simulink model "ev"  (R2021a)
settings: Solver=ode4  StartTime=0  StopTime=1082  FixedStep=sim_dt  RelTol=1e-3
model workspace (MAT data in the model file):
  T_eff_bp = [-270; -210; -150; -90; -30; 30; 90; 150; 210; 270]
  T_eff_bp_2 = [-270; -210; -150; -90; -30; 30; 90; 150; 210; 270]
  losses_table = [108927.107777 7820.2782368 7820.17609997 7820.2782368 7820.2782368 7820.2782368 7820.2782368 7820.26172359 7820.2782368 9345.38006027 108927.107777 7820.2782368 ... (100 elements, 10x10)]
  losses_table_2 = [108927.107777 7820.2782368 7820.17609997 7820.2782368 7820.2782368 7820.2782368 7820.2782368 7820.26172359 7820.2782368 9345.38006027 108927.107777 7820.2782368 ... (100 elements, 10x10)]
  w_eff_bp = [0; 888.888888889; 1777.77777778; 2666.66666667; 3555.55555556; 4444.44444444; 5333.33333333; 6222.22222222; 7111.11111111; 8000]
  w_eff_bp_2 = [0; 888.888888889; 1777.77777778; 2666.66666667; 3555.55555556; 4444.44444444; 5333.33333333; 6222.22222222; 7111.11111111; 8000]
undefined symbols (not defined in the file): Af, alpha, Bt, C, C_fa, C_free, C_sa_bat, C_sa_uc, Cd, Cmax, Continuous, Crr, DoD, effi, etaFD, etaG, FD, G, gear, Iucmax, m, M1m, M2m, Max, npar, npar_free, npara, nparf, nparfa, nparsa_bat, nparsa_UC, nser, nser_free, nserfa, nsersa_bat, nsersa_UC, Qbat, regenmax, Ri_BP, RL, ro, Rsc, Rsc_A, Rsc_F, Rsc_sa_bat, Rsc_sa_uc, rw, sim_dt, SOC_BP, SoCbatmax, SoCbatmin, SoCucmax, SoCucmin, speed, torque, VinBat, Voc_BP, Vuc, Vuc_fa, Vuc_free ... (+2)
libraries: autolibshared x41, simulink x26, autolibdcdc x13, autolibdatasheetbattery x7, autolibmappedmotor x6, fl_lib x3, nesl_utility x3, spsSupercapacitorLib x3, pid_lib x1
(part 7 of 18)

== system ev/Tesis/HESS/Battery model ==
  motor_pwr_contr : Inport
  Add : Sum  Inputs=+-
  Bus Selector : BusSelector  OutputSignals=BattSoc,BattCurr,BattPwr
  Compare To Constant1 : simulink/Logic and Bit Operations/Compare To Constant  relop=<=  const=0.2  OutDataTypeStr=boolean
  Constant2 : Constant  Value=293.15
  Current_calc : Product  Inputs=/*
  Datasheet Battery : autolibdatasheetbattery/Datasheet Battery  CapacityCtrl=Parameter  OutputVlt=Unfiltered  BattChargeMax=Qbat  Em=Voc_BP  CapLUTBp=SOC_BP  RInt=iR_bp  BattTempBp=Temp_bp  CapSOCBp=SOC_BP  Ns=nser  Np=npar  BattCapInit=Qbat*(1-DoD)  Tc=0.01  Vinit=3.3342*nser  RefBlkName='autolibdatasheetbattery/Datasheet Battery'
      settings: SourceProductBaseCode=PW
  Display1 : DisplayBlock  LabelPosition=Hide  Format=short  Transparency=1
  Gain4 : Gain  Gain=nser
  Gain5 : Gain  Gain=nser/npar
  MATLAB Function1 : MATLAB Function  TreatAsAtomicUnit=on
  Mux : Mux
  Mux12 : Mux  Inputs=2
  OCV1 : Lookup_n-D  NumberOfTableDimensions=1  BreakpointsForDimension1=SOC_BP  Table=Voc_BP  InternalRulePriority=Speed  RndMeth=Simplest  InputSameDT=on
  Product1 : Product
  Ri1 : Lookup_n-D  NumberOfTableDimensions=1  BreakpointsForDimension1=SOC_BP  Table=Ri_BP  InternalRulePriority=Speed  RndMeth=Simplest  InputSameDT=on
  Scope{1,5..7,13..14,26,39,44} (9 alike) : Scope
  Stop Simulation : Stop
  To Workspace9 : ToWorkspace  VariableName=Batt  SaveFormat=Structure With Time  SampleTime=-1
  <BattCurr> : Outport
  Voltage : Outport  Port=2
  wires:
  Bus Selector/2 -> <BattCurr>/1, Scope26/1, Product1/2  "<BattCurr>"
  Gain5/1 -> MATLAB Function1/1(Ri), Product1/1, Scope1/1
  Datasheet Battery/2 -> Voltage/1, Mux/2  "Voltage"
  Bus Selector/1 -> Compare To Constant1/1, Ri1/1, OCV1/1, Scope7/1  "<BattSoc>"
  Mux/1 -> Scope14/1
  Compare To Constant1/1 -> Scope5/1, Stop Simulation/1
  Gain4/1 -> Add/1, Mux/1, Current_calc/1
  OCV1/1 -> Gain4/1
  Bus Selector/3 -> Mux12/1  "<BattPwr>"
  Ri1/1 -> Gain5/1
  Add/1 -> Mux/3
  MATLAB Function1/1(Vb) -> Mux/4, Scope44/1
  Product1/1 -> Add/2
  Mux12/1 -> Scope39/1
  Datasheet Battery/1 -> Scope6/1, Bus Selector/1, To Workspace9/1
  Constant2/1 -> Datasheet Battery/2
  Current_calc/1 -> MATLAB Function1/2(Ib), Datasheet Battery/1, Scope13/1  "I_batt"
  motor_pwr_contr/1 -> Mux12/2, MATLAB Function1/3(Pmot), Current_calc/2

== system ev/Tesis/HESS/Battery with DC//DC ==
  motor_pwr_contr : Inport
  Add3 : Sum  Inputs=+-
  Bidirectional DC-DC2 : autolibdcdc/Bidirectional DC-DC  Tc=1/1000  Vinit=320  Plimit=100000  param_loss=Single efficiency measurement  eff=100  v_loss_bp=[0 200 400 600 800 1000]  i_loss_bp=[0 25 50 75 100]  losses_table=[100 100 100 100 100;100 150 200 250 300;100 200 300 400 500;100 250 400 550 700;100 300 500 700 900;100 350 600 850 1100]  v_eff_bp=[200 400 600 800 1000]  i_eff_bp=[25 50 75 100]  efficiency_table=[96.2 98.1 98.7 99;98.1 99 99.4 99.5;98.7 99.4 99.6 99.7;99 99.5 99.7 99.8;99.2 99.6 99.7 99.8]  x_v_bp=[-1000 -800 -600 -400 -200 200 400 600 800 1000]  x_i_bp=[-100 -75 -50 -25 25 50 75 100]  x_losses_mat=[200.400801603196 225.67703109328 200.803212851408 201.612903225806 199.999999999997 200 225 200;160.320641282556 180.541624874624 201.005025125625 202.020202020203 200 200 180 160;180.541624874624 180.722891566267 181.086519114686 197.568389057748 194.999999999999 179.999999999997 180 180;201.005025125625 181.086519114686 202.020202020203 193.67991845056 190 200 179.999999999997 200;202.020202020203 197.568389057748 193.67991845056 197.505197505197 190 190 194.999999999999 200;200 194.999999999999 190 190 197.505197505197 193.67991845056 197.568389057748 202.020202020203;200 179.999999999997 200 190 193.67991845056 202.020202020203 181.086519114686 201.005025125625;180 180 179.999999999997 194.999999999999 197.568389057748 181.086519114686 180.722891566267 180.541624874624;160 180 200 200 202.020202020203 201.005025125625 180.541624874624 160.320641282556;200 225 200 199.999999999997 201.612903225806 200.803212851408 225.67703109328 200.400801603196]  RefBlkName='autolibdcdc/Bidirectional DC-DC'
      settings: SourceProductBaseCode=PW
  Bus Selector2 : BusSelector  OutputSignals=BattSoc,BattCurr,BattPwr
  Bus Selector3 : BusSelector  OutputSignals=SrcPwr,LdPwr
  Compare To Constant3 : simulink/Logic and Bit Operations/Compare To Constant  relop=<=  const=0.2  OutDataTypeStr=boolean
  Constant10 : Constant  Value=320
  Constant9 : Constant  Value=293.15
  Current_calc1 : Product  Inputs=/*
  Datasheet Battery2 : autolibdatasheetbattery/Datasheet Battery  CapacityCtrl=Parameter  OutputVlt=Unfiltered  BattChargeMax=Qbat  Em=Voc_BP  CapLUTBp=SOC_BP  RInt=iR_bp  BattTempBp=Temp_bp  CapSOCBp=SOC_BP  Ns=nser  Np=npar  BattCapInit=Qbat*(1-DoD)  Tc=0.01  Vinit=3.3342*nser  RefBlkName='autolibdatasheetbattery/Datasheet Battery'
      settings: SourceProductBaseCode=PW
  Display3 : DisplayBlock  LabelPosition=Hide  Format=short  Transparency=1
  Divide : Product  Inputs=*/
  Gain10 : Gain  Gain=nser/npar
  Gain8 : Gain
  Gain9 : Gain  Gain=nser
  Mux10 : Mux
  Mux4 : Mux  Inputs=3
  Mux9 : Mux  Inputs=2
  OCV3 : Lookup_n-D  NumberOfTableDimensions=1  BreakpointsForDimension1=SOC_BP  Table=Voc_BP  InternalRulePriority=Speed  RndMeth=Simplest  InputSameDT=on
  Product3 : Product
  Ri3 : Lookup_n-D  NumberOfTableDimensions=1  BreakpointsForDimension1=SOC_BP  Table=Ri_BP  InternalRulePriority=Speed  RndMeth=Simplest  InputSameDT=on
  Scope{1,27..37} (12 alike) : Scope
  Stop Simulation2 : Stop
  To Workspace2 : ToWorkspace  VariableName=Batt3  SaveFormat=Structure With Time  SampleTime=-1
  wires:
  OCV3/1 -> Gain9/1
  Compare To Constant3/1 -> Scope31/1, Stop Simulation2/1
  Bus Selector2/1 -> Compare To Constant3/1, Ri3/1, OCV3/1, Scope33/1  "<BattSoc>"
  Mux9/1 -> Scope30/1
  motor_pwr_contr/1 -> Gain8/1, Mux10/3
  Bus Selector2/3 -> Scope37/1, Mux10/4  "<BattPwr>"
  Current_calc1/1 -> Scope28/1, Bidirectional DC-DC2/3  "I_batt"
  Constant9/1 -> Datasheet Battery2/2
  Bus Selector3/1 -> Mux10/1  "<SrcPwr>"
  Bidirectional DC-DC2/1 -> Bus Selector3/1
  Bus Selector3/2 -> Mux10/2  "<LdPwr>"
  Gain9/1 -> Bidirectional DC-DC2/2, Add3/1, Mux4/1
  Add3/1 -> Mux4/3
  Mux10/1 -> Scope36/1
  Constant10/1 -> Bidirectional DC-DC2/1
  Product3/1 -> Add3/2
  Gain8/1 -> Current_calc1/2
  Gain10/1 -> Product3/1, Scope27/1
  Datasheet Battery2/2 -> Mux4/2  "Voltage"
  Datasheet Battery2/1 -> Scope32/1, Bus Selector2/1, To Workspace2/1
  Bus Selector2/2 -> Product3/2  "<BattCurr>"
  Mux4/1 -> Scope29/1
  Ri3/1 -> Gain10/1
  Bidirectional DC-DC2/2 -> Divide/1, Current_calc1/1, Scope34/1
  Bidirectional DC-DC2/3 -> Datasheet Battery2/1, Mux9/1
  Divide/1 -> Scope1/1

== system ev/Tesis/HESS/Capacitor ideal ==
  motor_pwr_contr : Inport
  C*(V^2)/2 : Product  Inputs=**/
  Constant1 : Constant  Value=0
  Constant11 : Constant  Value=C
  Constant12 : Constant  Value=2
  Current_calc2 : Product  Inputs=/*
  Derivative : Derivative
  Divide : Product  Inputs=*/
  Gain12 : Gain  Gain=-1/3600
  Gain14 : Gain  Gain=-1
  Gain21 : Gain  Gain=-1
  Integrator1 : Integrator  InitialCondition=Vuc
  Integrator3 : Integrator
  Mux15 : Mux  Inputs=3
  POW Wh1 : Scope
  Scope{41,46..47,59} (4 alike) : Scope
  Square : Math  Operator=square  SaturateOnIntegerOverflow=on
  Switch17 : Switch  Threshold=VinBat*nser*3*Qbat*npar
  Switch18 : Switch  Threshold=-VinBat*nser*3*Qbat*npar
  Switch19 : Switch
  energy Wh : Scope
  wires:
  Gain12/1 -> energy Wh/1
  Switch19/1 -> Scope46/1, Current_calc2/2  "Pow"
  Switch17/1 -> Mux15/2, Switch19/1  "Pow"
  C*(V^2)/2/1 -> Derivative/1, Gain12/1
  Mux15/1 -> Scope47/1
  Constant11/1 -> Gain21/1, C*(V^2)/2/2
  motor_pwr_contr/1 -> Mux15/1, Switch19/2, Switch18/3, Switch18/2, Switch17/1, Switch17/2
  Integrator3/1 -> Square/1
  Switch18/1 -> Switch19/3, Mux15/3  "Pow"
  Derivative/1 -> Gain14/1
  Constant1/1 -> Switch18/1, Switch17/3
  Integrator1/1 -> Current_calc2/1, Scope59/1
  Constant12/1 -> C*(V^2)/2/3
  Divide/1 -> Integrator3/1, Integrator1/1
  Current_calc2/1 -> Divide/1, Scope41/1  "I_batt"
  Square/1 -> C*(V^2)/2/1
  Gain21/1 -> Divide/2
  Gain14/1 -> POW Wh1/1

== system ev/Tesis/HESS/Capacitor real ==
  motor_pwr_contr : Inport
  Add4 : Sum
  Add5 : Sum
  Constant13 : Constant  Value=0
  Current_calc3 : Product  Inputs=/*
  Gain15 : Gain  Gain=1/(C*RL)
  Gain16 : Gain  Gain=-Rsc
  Gain17 : Gain  Gain=C/2
  Gain18 : Gain  Gain=0.6
  Gain19 : Gain  Gain=1/(Vuc*Vuc)
  Gain3 : Gain  Gain=-1/C
  Integrator5 : Integrator  InitialCondition=Vuc
  Math Function : Math  Operator=square  SaturateOnIntegerOverflow=on
  Math Function1 : Math  Operator=square  SaturateOnIntegerOverflow=on
  Mux16 : Mux  Inputs=3
  Scope{48..51} (4 alike) : Scope
  Scope52 : Scope  Commented=on
  Switch14 : Switch  Threshold=VinBat*nser*3*Qbat*npar
  Switch15 : Switch  Threshold=-VinBat*nser*3*Qbat*npar
  Switch16 : Switch
  wires:
  Switch16/1 -> Scope50/1, Current_calc3/2  "Pow"
  Current_calc3/1 -> Gain16/1, Gain3/1  "I_uc"
  Add4/1 -> Integrator5/1  "dVc/dt"
  motor_pwr_contr/1 -> Mux16/1, Switch16/2, Switch15/3, Switch15/2, Switch14/1, Switch14/2
  Mux16/1 -> Scope51/1
  Integrator5/1 -> Add5/1, Gain18/1, Math Function/1, Gain15/1  "Vc"
  Switch15/1 -> Switch16/3, Mux16/3  "Pow"
  Gain15/1 -> Add4/1
  Switch14/1 -> Mux16/2, Switch16/1  "Pow"
  Constant13/1 -> Switch15/1, Switch14/3
  Math Function/1 -> Gain17/1
  Gain16/1 -> Add5/2  "i/C"
  Math Function1/1 -> Gain19/1
  Gain17/1 -> Scope48/1
  Gain18/1 -> Math Function1/1
  Add5/1 -> Scope49/1, Current_calc3/1  "dVc/dt"
  Gain19/1 -> Scope52/1
  Gain3/1 -> Add4/2  "i/C"

== system ev/Tesis/HESS/Capacitor semi ideal ==
  motor_pwr_contr : Inport
  Add7 : Sum  Inputs=+-
  Bidirectional DC-DC1 : autolibdcdc/Bidirectional DC-DC  Tc=1/1000  Vinit=320  Plimit=100000  param_loss=Single efficiency measurement  eff=95  v_loss_bp=[0 200 400 600 800 1000]  i_loss_bp=[0 25 50 75 100]  losses_table=[100 100 100 100 100;100 150 200 250 300;100 200 300 400 500;100 250 400 550 700;100 300 500 700 900;100 350 600 850 1100]  v_eff_bp=[200 400 600 800 1000]  i_eff_bp=[25 50 75 100]  efficiency_table=[96.2 98.1 98.7 99;98.1 99 99.4 99.5;98.7 99.4 99.6 99.7;99 99.5 99.7 99.8;99.2 99.6 99.7 99.8]  x_v_bp=[-1000 -800 -600 -400 -200 200 400 600 800 1000]  x_i_bp=[-100 -75 -50 -25 25 50 75 100]  x_losses_mat=[200.400801603196 225.67703109328 200.803212851408 201.612903225806 199.999999999997 200 225 200;160.320641282556 180.541624874624 201.005025125625 202.020202020203 200 200 180 160;180.541624874624 180.722891566267 181.086519114686 197.568389057748 194.999999999999 179.999999999997 180 180;201.005025125625 181.086519114686 202.020202020203 193.67991845056 190 200 179.999999999997 200;202.020202020203 197.568389057748 193.67991845056 197.505197505197 190 190 194.999999999999 200;200 194.999999999999 190 190 197.505197505197 193.67991845056 197.568389057748 202.020202020203;200 179.999999999997 200 190 193.67991845056 202.020202020203 181.086519114686 201.005025125625;180 180 179.999999999997 194.999999999999 197.568389057748 181.086519114686 180.722891566267 180.541624874624;160 180 200 200 202.020202020203 201.005025125625 180.541624874624 160.320641282556;200 225 200 199.999999999997 201.612903225806 200.803212851408 225.67703109328 200.400801603196]  RefBlkName='autolibdcdc/Bidirectional DC-DC'
      settings: SourceProductBaseCode=PW
  Constant14 : Constant  Value=0
  Constant15 : Constant  Value=320
  Current_calc4 : Product  Inputs=/*
  Gain20 : Gain  Gain=Rsc
  Gain22 : Gain  Gain=C/2
  Gain23 : Gain
  Gain24 : Gain  Gain=1/(Vuc*Vuc)
  Gain25 : Gain  Gain=-1/C
  Integrator6 : Integrator  InitialCondition=Vuc*0.2
  Math Function2 : Math  Operator=square  SaturateOnIntegerOverflow=on
  Math Function3 : Math  Operator=square  SaturateOnIntegerOverflow=on
  Mux17 : Mux  Inputs=3
  Scope{53..58,60} (7 alike) : Scope
  Switch20 : Switch  Threshold=VinBat*nser*3*Qbat*npar
  Switch21 : Switch  Threshold=-VinBat*nser*3*Qbat*npar
  Switch22 : Switch
  Info : Outport
  wires:
  Switch21/1 -> Switch22/3, Mux17/3  "-Pow"
  motor_pwr_contr/1 -> Mux17/1, Switch22/2, Switch21/3, Switch21/2, Switch20/1, Switch20/2
  Constant14/1 -> Switch21/1, Switch20/3
  Current_calc4/1 -> Bidirectional DC-DC1/3  "I_uc"
  Switch22/1 -> Scope55/1, Current_calc4/2  "Pow"
  Switch20/1 -> Mux17/2, Switch22/1  "+Pow"
  Gain22/1 -> Scope53/1
  Gain23/1 -> Math Function3/1
  Integrator6/1 -> Gain23/1, Math Function2/1, Add7/1  "Vc"
  Bidirectional DC-DC1/2 -> Current_calc4/1
  Mux17/1 -> Scope56/1
  Gain24/1 -> Scope57/1
  Add7/1 -> Scope54/1, Bidirectional DC-DC1/2
  Constant15/1 -> Bidirectional DC-DC1/1
  Gain20/1 -> Add7/2, Scope60/1  "i*Rs"
  Math Function2/1 -> Gain22/1
  Gain25/1 -> Integrator6/1  "i/C"
  Bidirectional DC-DC1/3 -> Gain25/1, Gain20/1, Scope58/1
  Math Function3/1 -> Gain24/1
  Bidirectional DC-DC1/1 -> Info/1

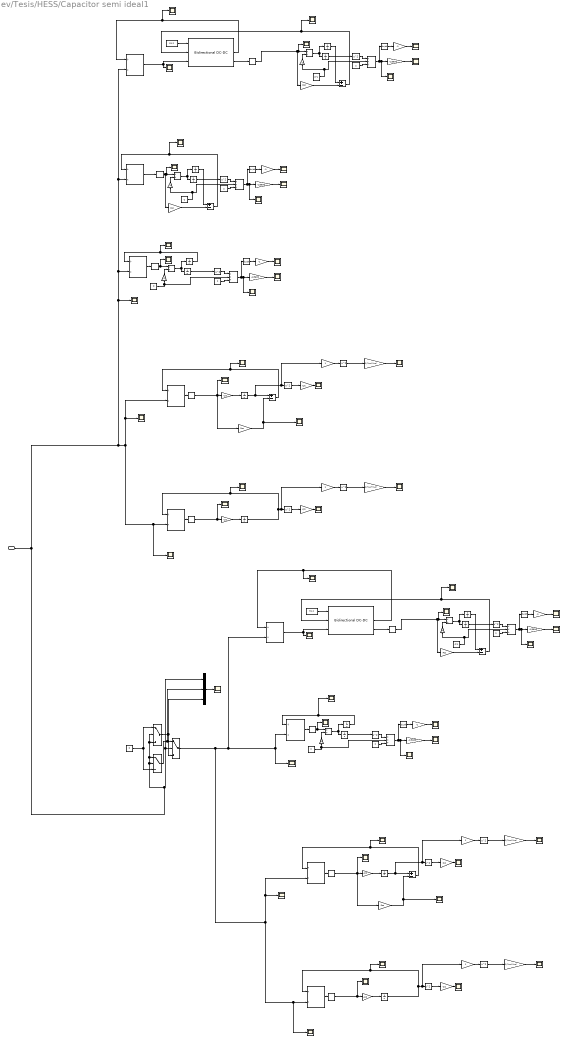
== system ev/Tesis/HESS/Capacitor semi ideal1 ==
  motor_pwr_contr : Inport
  Add{1..4,7} (5 alike) : Sum  Inputs=+-
  Bidirectional DC-DC1 : autolibdcdc/Bidirectional DC-DC  Tc=1/1000  Vinit=51.2  Plimit=100000  param_loss=Single efficiency measurement  eff=95  v_loss_bp=[0 200 400 600 800 1000]  i_loss_bp=[0 25 50 75 100]  losses_table=[100 100 100 100 100;100 150 200 250 300;100 200 300 400 500;100 250 400 550 700;100 300 500 700 900;100 350 600 850 1100]  v_eff_bp=[200 400 600 800 1000]  i_eff_bp=[25 50 75 100]  efficiency_table=[96.2 98.1 98.7 99;98.1 99 99.4 99.5;98.7 99.4 99.6 99.7;99 99.5 99.7 99.8;99.2 99.6 99.7 99.8]  x_v_bp=[-1000 -800 -600 -400 -200 200 400 600 800 1000]  x_i_bp=[-100 -75 -50 -25 25 50 75 100]  x_losses_mat=[200.400801603196 225.67703109328 200.803212851408 201.612903225806 199.999999999997 200 225 200;160.320641282556 180.541624874624 201.005025125625 202.020202020203 200 200 180 160;180.541624874624 180.722891566267 181.086519114686 197.568389057748 194.999999999999 179.999999999997 180 180;201.005025125625 181.086519114686 202.020202020203 193.67991845056 190 200 179.999999999997 200;202.020202020203 197.568389057748 193.67991845056 197.505197505197 190 190 194.999999999999 200;200 194.999999999999 190 190 197.505197505197 193.67991845056 197.568389057748 202.020202020203;200 179.999999999997 200 190 193.67991845056 202.020202020203 181.086519114686 201.005025125625;180 180 179.999999999997 194.999999999999 197.568389057748 181.086519114686 180.722891566267 180.541624874624;160 180 200 200 202.020202020203 201.005025125625 180.541624874624 160.320641282556;200 225 200 199.999999999997 201.612903225806 200.803212851408 225.67703109328 200.400801603196]  RefBlkName='autolibdcdc/Bidirectional DC-DC'
      settings: SourceProductBaseCode=PW
  Bidirectional DC-DC2 : autolibdcdc/Bidirectional DC-DC  Tc=1/1000  Vinit=51.2  Plimit=100000  param_loss=Single efficiency measurement  eff=95  v_loss_bp=[0 200 400 600 800 1000]  i_loss_bp=[0 25 50 75 100]  losses_table=[100 100 100 100 100;100 150 200 250 300;100 200 300 400 500;100 250 400 550 700;100 300 500 700 900;100 350 600 850 1100]  v_eff_bp=[200 400 600 800 1000]  i_eff_bp=[25 50 75 100]  efficiency_table=[96.2 98.1 98.7 99;98.1 99 99.4 99.5;98.7 99.4 99.6 99.7;99 99.5 99.7 99.8;99.2 99.6 99.7 99.8]  x_v_bp=[-1000 -800 -600 -400 -200 200 400 600 800 1000]  x_i_bp=[-100 -75 -50 -25 25 50 75 100]  x_losses_mat=[200.400801603196 225.67703109328 200.803212851408 201.612903225806 199.999999999997 200 225 200;160.320641282556 180.541624874624 201.005025125625 202.020202020203 200 200 180 160;180.541624874624 180.722891566267 181.086519114686 197.568389057748 194.999999999999 179.999999999997 180 180;201.005025125625 181.086519114686 202.020202020203 193.67991845056 190 200 179.999999999997 200;202.020202020203 197.568389057748 193.67991845056 197.505197505197 190 190 194.999999999999 200;200 194.999999999999 190 190 197.505197505197 193.67991845056 197.568389057748 202.020202020203;200 179.999999999997 200 190 193.67991845056 202.020202020203 181.086519114686 201.005025125625;180 180 179.999999999997 194.999999999999 197.568389057748 181.086519114686 180.722891566267 180.541624874624;160 180 200 200 202.020202020203 201.005025125625 180.541624874624 160.320641282556;200 225 200 199.999999999997 201.612903225806 200.803212851408 225.67703109328 200.400801603196]  RefBlkName='autolibdcdc/Bidirectional DC-DC'
      settings: SourceProductBaseCode=PW
  C*(V^2)/(2)(a) : Product  Inputs=**/
  C*(V^2)/2 : Product  Inputs=**/
  C*(V^2)/2(1) : Product  Inputs=**/
  C*(V^2)/2(1)1 : Product  Inputs=**/
  C*(V^2)/2(1)2 : Product  Inputs=**/
  Constant1 : Constant  Value=0
  Constant{3,5,7,10,12} (5 alike) : Constant  Value=2
  Constant11 : Constant  Value=C
  Constant13 : Constant  Value=51.2
  Constant2 : Constant  Value=C
  Constant4 : Constant  Value=C
  Constant6 : Constant  Value=C*1
  Constant8 : Constant  Value=C*1
  Constant9 : Constant  Value=51.2
  Current_calc{1..9} (9 alike) : Product  Inputs=/*
  Derivative{,1..4} (5 alike) : Derivative
  Divide{,1..4} (5 alike) : Product  Inputs=*/
  Gain{1..2,7,22} (4 alike) : Gain  Gain=C/2
  Gain{5,10,15,25} (4 alike) : Gain  Gain=-1/C
  Gain{3,8,11,23} (4 alike) : Gain
  Gain{12,16,19,29,33} (5 alike) : Gain  Gain=-1/3600
  Gain{4,9,13,24} (4 alike) : Gain  Gain=1/(Vuc*Vuc)
  Gain{14,17..18,21,26..27,30..31,34..35} (10 alike) : Gain  Gain=-1
  Gain{6,20,28,32,36} (5 alike) : Gain  Gain=Rsc
  Integrator{1,6..7,9} (4 alike) : Integrator  InitialCondition=Vuc*10
  Integrator{3,8,10..11,13} (5 alike) : Integrator
  Integrator12 : Integrator  InitialCondition=Vuc*1
  Integrator14 : Integrator  InitialCondition=Vuc*1
  Integrator2 : Integrator  InitialCondition=Vuc
  Integrator4 : Integrator  InitialCondition=Vuc
  Integrator5 : Integrator  InitialCondition=Vuc
  Math Function{1..8} (8 alike) : Math  Operator=square  SaturateOnIntegerOverflow=on
  Memory{,1..8} (9 alike) : Memory
  Mux15 : Mux  Inputs=3
  POW Wh{1..5} (5 alike) : Scope
  Scope{1..30,41,46..47,53..55,57,59..60} (39 alike) : Scope
  Square{,1..4} (5 alike) : Math  Operator=square  SaturateOnIntegerOverflow=on
  Switch17 : Switch  Threshold=VinBat*nser*1*Qbat*npar
  Switch18 : Switch  Threshold=-VinBat*nser*1*Qbat*npar
  Switch19 : Switch
  energy{,1..4} (5 alike) : Scope
  energy Wh{,1..4} (5 alike) : Scope
  wires:
  Gain22/1 -> Scope53/1
  Gain23/1 -> Math Function3/1
  Integrator6/1 -> Gain23/1, Math Function2/1, Add7/1  "Vc"
  Gain24/1 -> Scope57/1
  Add7/1 -> Current_calc4/1, Scope54/1
  Gain20/1 -> Add7/2, Scope60/1  "i*Rs"
  Math Function2/1 -> Gain22/1
  Gain25/1 -> Integrator6/1  "i/C"
  Current_calc4/1 -> Memory/1
  Math Function3/1 -> Gain24/1
  Memory/1 -> Scope2/1, Gain20/1, Gain25/1
  Current_calc1/1 -> Memory1/1
  Math Function4/1 -> Gain4/1
  Gain2/1 -> Scope3/1
  Gain5/1 -> Integrator1/1  "i/C"
  Memory1/1 -> Scope1/1, Gain5/1
  Gain4/1 -> Scope6/1
  Integrator1/1 -> Current_calc1/1, Scope4/1, Gain3/1, Math Function1/1  "Vc"
  Gain3/1 -> Math Function4/1
  Math Function1/1 -> Gain2/1
  Square/1 -> C*(V^2)/2/1
  Gain21/1 -> Divide/2
  Gain14/1 -> POW Wh1/1
  Switch17/1 -> Mux15/2, Switch19/1  "limit max"
  Constant1/1 -> Switch18/1, Switch17/3
  Integrator2/1 -> Current_calc2/1, Scope59/1
  Constant11/1 -> Gain21/1, C*(V^2)/2/2
  Derivative/1 -> Gain14/1
  Constant12/1 -> C*(V^2)/2/3
  Switch18/1 -> Switch19/3, Mux15/3  "limit min"
  Divide/1 -> Integrator3/1, Integrator2/1
  Mux15/1 -> Scope47/1
  Integrator3/1 -> Square/1
  Current_calc2/1 -> Memory4/1  "I_batt"
  C*(V^2)/2/1 -> Derivative/1, energy/1, Gain12/1
  Switch19/1 -> Scope11/1, Current_calc3/2, Current_calc5/2, Scope14/1, Current_calc9/2, Scope46/1, Current_calc2/2  "Pow"
  Gain12/1 -> energy Wh/1
  Current_calc5/1 -> Memory2/1
  Gain11/1 -> Math Function8/1
  Math Function5/1 -> Gain1/1
  Integrator4/1 -> Current_calc3/1, Scope10/1, Gain11/1, Math Function5/1  "Vc"
  Gain1/1 -> Scope9/1
  Gain15/1 -> Integrator4/1  "i/C"
  Math Function8/1 -> Gain13/1
  Current_calc3/1 -> Memory3/1
  Add1/1 -> Current_calc5/1, Scope13/1
  Math Function7/1 -> Gain9/1
  Gain7/1 -> Scope12/1
  Gain13/1 -> Scope16/1
  Gain10/1 -> Integrator5/1  "i/C"
  Memory2/1 -> Scope8/1, Gain6/1, Gain10/1
  Gain6/1 -> Add1/2, Scope17/1  "i*Rs"
  Gain9/1 -> Scope15/1
  Integrator5/1 -> Gain8/1, Math Function6/1, Add1/1  "Vc"
  Memory3/1 -> Scope7/1, Gain15/1
  Gain8/1 -> Math Function7/1
  Math Function6/1 -> Gain7/1
  Memory4/1 -> Divide/1, Scope41/1
  C*(V^2)/(2)(a)/1 -> Derivative1/1, energy1/1, Gain16/1
  Gain16/1 -> energy Wh1/1
  Current_calc6/1 -> Memory6/1  "I_batt"
  Integrator8/1 -> Square1/1
  Constant3/1 -> C*(V^2)/(2)(a)/3
  Derivative1/1 -> Gain17/1
  Divide1/1 -> Integrator8/1, Integrator7/1
  Integrator7/1 -> Current_calc6/1, Scope20/1
  Gain17/1 -> POW Wh2/1
  Gain18/1 -> Divide1/2
  Constant2/1 -> Gain18/1, C*(V^2)/(2)(a)/2
  Square1/1 -> C*(V^2)/(2)(a)/1
  Constant4/1 -> Gain27/1, C*(V^2)/2(1)/2
  Square2/1 -> C*(V^2)/2(1)/1
  Gain27/1 -> Divide2/2
  Gain26/1 -> POW Wh3/1
  Divide2/1 -> Integrator10/1, Integrator9/1
  Integrator10/1 -> Square2/1
  Derivative2/1 -> Gain26/1
  Constant5/1 -> C*(V^2)/2(1)/3
  C*(V^2)/2(1)/1 -> Derivative2/1, energy2/1, Gain19/1
  Gain19/1 -> energy Wh2/1
  Current_calc7/1 -> Memory5/1  "I_batt"
  Gain28/1 -> Add2/2  "i*Rs"
  Integrator9/1 -> Add2/1  "UC internal voltage"
  Add2/1 -> Scope23/1, Current_calc7/1  "voltage"
  Memory6/1 -> Divide1/1, Scope18/1
  Memory5/1 -> Gain28/1, Divide2/1, Scope21/1
  motor_pwr_contr/1 -> Mux15/1, Switch19/2, Switch18/3, Switch18/2, Switch17/1, Switch17/2, Current_calc6/2, Current_calc8/2, Current_calc7/2, Scope19/1, Scope5/1, Current_calc1/2, Current_calc4/2, Scope55/1  "limited Pow"
  Bidirectional DC-DC2/2 -> Scope26/1, Current_calc8/1
  Divide3/1 -> Integrator11/1, Integrator12/1
  Add3/1 -> Bidirectional DC-DC2/2, Scope25/1  "voltage"
  Gain30/1 -> POW Wh4/1
  Bidirectional DC-DC2/3 -> Memory7/1  "I_batt"
  Gain32/1 -> Add3/2  "i*Rs"
  C*(V^2)/2(1)1/1 -> Derivative3/1, energy3/1, Gain29/1
  Gain29/1 -> energy Wh3/1
  Derivative3/1 -> Gain30/1
  Integrator11/1 -> Square3/1
  Integrator12/1 -> Add3/1  "UC internal voltage"
  Square3/1 -> C*(V^2)/2(1)1/1
  Constant6/1 -> Gain31/1, C*(V^2)/2(1)1/2
  Gain31/1 -> Divide3/2
  Constant7/1 -> C*(V^2)/2(1)1/3
  Constant9/1 -> Bidirectional DC-DC2/1
  Current_calc8/1 -> Bidirectional DC-DC2/3, Scope22/1
  Memory7/1 -> Gain32/1, Divide3/1, Scope24/1
  Bidirectional DC-DC1/3 -> Memory8/1  "I_batt"
  Constant10/1 -> C*(V^2)/2(1)2/3
  Integrator13/1 -> Square4/1
  Square4/1 -> C*(V^2)/2(1)2/1
  Constant8/1 -> Gain35/1, C*(V^2)/2(1)2/2
  C*(V^2)/2(1)2/1 -> Derivative4/1, energy4/1, Gain33/1
  Derivative4/1 -> Gain34/1
  Current_calc9/1 -> Bidirectional DC-DC1/3, Scope27/1
  Gain33/1 -> energy Wh4/1
  Gain36/1 -> Add4/2  "i*Rs"
  Integrator14/1 -> Add4/1  "UC internal voltage"
  Bidirectional DC-DC1/2 -> Scope30/1, Current_calc9/1
  Add4/1 -> Bidirectional DC-DC1/2, Scope29/1  "voltage"
  Gain34/1 -> POW Wh5/1
  Gain35/1 -> Divide4/2
  Divide4/1 -> Integrator13/1, Integrator14/1
  Memory8/1 -> Gain36/1, Divide4/1, Scope28/1
  Constant13/1 -> Bidirectional DC-DC1/1

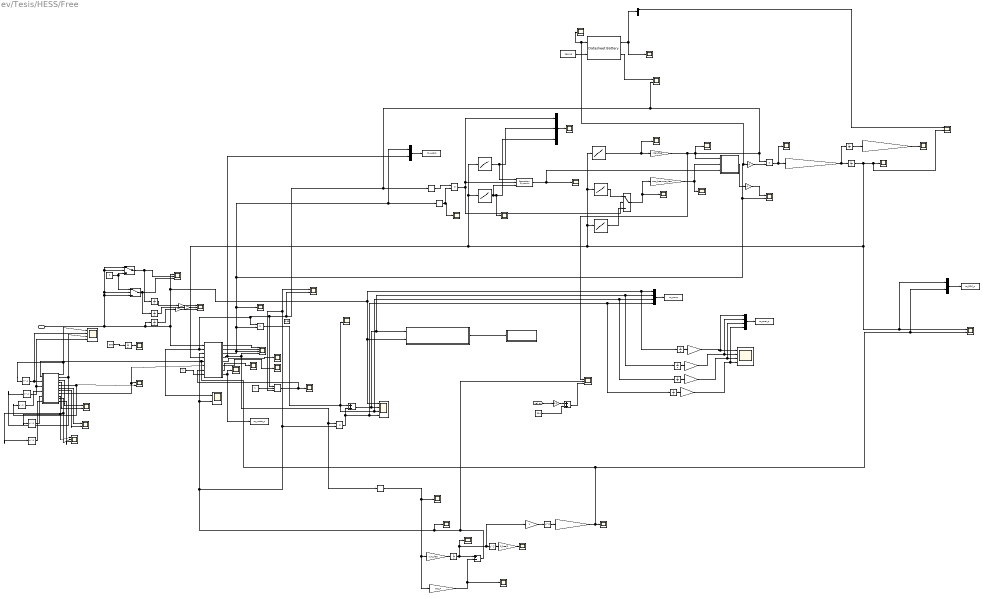
== system ev/Tesis/HESS/Free ==
  motor_pwr_contr : Inport
  Add : Sum
  Add1 : Sum  Inputs=+-
  Add2 : Sum
  Bus Selector : BusSelector  OutputSignals=BattSoc,BattCurr,BattPwr
  Constant : Constant  Value=304
  Constant1 : Constant
  Constant2 : Constant  Value=500
  Constant3 : Constant  Value=0.95
  Constant4 : Constant
  Constant5 : Constant  Value=0
  Constant6 : Constant  Value=293.15
  Datasheet Battery : autolibdatasheetbattery/Datasheet Battery  CapacityCtrl=Parameter  OutputVlt=Unfiltered  BattChargeMax=Qbat  Em=Voc_BP  CapLUTBp=SOC_BP  RInt=iR_bp  BattTempBp=Temp_bp  CapSOCBp=SOC_BP  Ns=nser_free  Np=npar_free  BattCapInit=Qbat*(1-DoD)  Tc=0.01  Vinit=3.3342*nser  RefBlkName='autolibdatasheetbattery/Datasheet Battery'
      settings: SourceProductBaseCode=PW
  Delay{1..5} (5 alike) : Delay  DelayLength=1  InitialCondition=0
  Divide1 : Product  Inputs=**/
  Gain : Gain  Gain=nser_free
  Gain1 : Gain  Gain=Rsc_F
  Gain10 : Gain  Gain=0.1
  Gain11 : Gain  Gain=(Qbat*VinBat*nser_free*npar_free)
  Gain{12..15} (4 alike) : Gain  Gain=1/(3600)
  Gain16 : Gain  Gain=1/3600
  Gain17 : Gain  Gain=1/3600
  Gain18 : Gain  Gain=1/3600
  Gain2 : Gain  Gain=C_free/2
  Gain3 : Gain
  Gain4 : Gain  Gain=1/(Vuc_free*Vuc_free)
  Gain5 : Gain  Gain=-1/C_free
  Gain6 : Gain  Gain=nser_free/npar_free
  Gain7 : Gain  Gain=1/(Qbat*VinBat*nser_free*npar_free*3600)
  Gain8 : Gain  Gain=-1
  Gain9 : Gain  Gain=-1
  Ibatt1 : Scope  NumInputPorts=2
  Integrator{,1,3..9} (9 alike) : Integrator
  Integrator2 : Integrator  InitialCondition=Vuc_free*0.95  UpperSaturationLimit=Vuc  LowerSaturationLimit=Vuc*0
  MATLAB Function : MATLAB Function  TreatAsAtomicUnit=on
  MATLAB Function1 : MATLAB Function  TreatAsAtomicUnit=on
  MATLAB Function2 : MATLAB Function  TreatAsAtomicUnit=on
  Math Function1 : Math  Operator=square  SaturateOnIntegerOverflow=on
  Math Function4 : Math  Operator=square  SaturateOnIntegerOverflow=on
  Memory : Memory
  Memory1 : Memory
  Memory2 : Memory
  Mux1 : Mux
  Mux13 : Mux  Inputs=3
  Mux2 : Mux  Inputs=2
  Mux3 : Mux  Inputs=2
  Mux4 : Mux
  OCV : Lookup_n-D  NumberOfTableDimensions=1  BreakpointsForDimension1=SOC_BP  Table=Voc_BP  InternalRulePriority=Speed  RndMeth=Simplest  InputSameDT=on
  PMG_max : Lookup_n-D  NumberOfTableDimensions=1  BreakpointsForDimension1=SOC_BP  Table=Voc_BP*nser_free*3*Qbat*npar_free  InternalRulePriority=Speed  RndMeth=Simplest  InputSameDT=on
  PMG_min : Lookup_n-D  NumberOfTableDimensions=1  BreakpointsForDimension1=SOC_BP  Table=-Voc_BP*nser_free*3*Qbat*npar_free  InternalRulePriority=Speed  RndMeth=Simplest  InputSameDT=on
  Pow1 : Scope
  Product{,1..3} (4 alike) : Product
  Ri : Lookup_n-D  NumberOfTableDimensions=1  BreakpointsForDimension1=SOC_BP  Table=Ri_BP  InternalRulePriority=Speed  RndMeth=Simplest  InputSameDT=on
  Ri4 : Lookup_n-D  NumberOfTableDimensions=1  BreakpointsForDimension1=SOC_BP  Table=Ri_BP  InternalRulePriority=Speed  RndMeth=Simplest  InputSameDT=on
  SOC : Integrator  InitialCondition=(1-DoD)
  Saturation Dynamic : simulink/Discontinuities/Saturation Dynamic  OutMin=[]  OutMax=[]  OutDataTypeStr=Inherit: Same as second input  OutDataType=fixdt(1, 16)  OutScaling=2^-10  DoSatur=off
  Scope{1,6..7,9,11..12,14..16,42..43,53..54,57} (14 alike) : Scope
  Scope10 : Scope  NumInputPorts=4
  Scope{3,8,13,17..18} (5 alike) : Scope  NumInputPorts=2
  Scope2 : Scope  NumInputPorts=4
  Scope28 : Scope  NumInputPorts=4
  Scope4 : Scope  NumInputPorts=3
  Scope5 : Scope  NumInputPorts=3
  Scope55 : Scope  NumInputPorts=3
  SoC : Scope
  Subsystem : Subsystem
  Switch : Switch
  Switch1 : Switch
  Switch13 : Switch  Criteria=u2 > Threshold
  To Workspace : ToWorkspace  VariableName=zz_powp  SaveFormat=Structure With Time  SampleTime=-1
  To Workspace1 : ToWorkspace  VariableName=zz_SOC_p  SaveFormat=Structure With Time  SampleTime=-1
  To Workspace2 : ToWorkspace  VariableName=zz_mode_p  SaveFormat=Structure With Time  SampleTime=-1
  To Workspace3 : ToWorkspace  VariableName=zz_ener_p  SaveFormat=Structure With Time  SampleTime=-1
  To Workspace4 : ToWorkspace  VariableName=zz_I_pass  SaveFormat=Structure With Time  SampleTime=-1
  Vo : Scope
  Vo1 : Scope
  Voc : Scope
  Voltage : Scope  NumInputPorts=2
  ab : Scope  NumInputPorts=2
  ab1 : Scope  NumInputPorts=3
  ener Wh : Scope
  ener Wh2 : Scope  NumInputPorts=4
  error : Scope
  flag_pow : Scope
  iR : Scope
  iRt : Scope
  mod : Scope  NumInputPorts=2
  mode : Scope
  stop : Scope
  test : Scope  NumInputPorts=2
  vehicle dynamics : Subsystem
  wires:
  motor_pwr_contr/1 -> Switch1/3, Switch1/2, Switch/2, Switch/1, Integrator8/1, Integrator4/1, Mux1/1, Subsystem/2(motor_pwr_contr), Scope10/1, Scope55/1, MATLAB Function/1(Preq)  "Pow"
  MATLAB Function/2(Iout) -> Scope28/2  "Iout tot"
  MATLAB Function/5(err) -> error/1
  MATLAB Function/6(stop) -> stop/1
  MATLAB Function/7(flagpow) -> flag_pow/1
  MATLAB Function/8(mode) -> To Workspace2/1, mode/1
  Gain1/1 -> Add1/2, Scope14/1  "i*Rs"
  Gain2/1 -> Scope53/1
  Math Function4/1 -> Gain4/1
  Math Function1/1 -> Gain2/1
  Gain5/1 -> Integrator2/1
  Gain3/1 -> Math Function4/1
  MATLAB Function/4(I_uc) -> Mux3/2, Scope28/4, Memory/1, Product3/1  "I uc"
  Integrator2/1 -> Scope9/1, Gain3/1, Math Function1/1, Add1/1  "Vc"
  Memory/1 -> Gain1/1, Gain5/1, Scope54/1
  Add/1 -> Integrator5/1, Mux1/2, Subsystem/1(In1), Scope10/2
  PMG_max/1 -> Saturation Dynamic/1, Mux13/2
  Gain7/1 -> Integrator1/1, SOC/1
  PMG_min/1 -> Saturation Dynamic/3, Scope43/1, Mux13/3
  Product/1 -> Pow1/1, Gain7/1
  Saturation Dynamic/1 -> Vo1/1, MATLAB Function2/3(P)
  Gain11/1 -> ener Wh/1
  Switch13/1 -> Gain6/1, iR/1
  Integrator1/1 -> Gain11/1
  OCV/1 -> Vo/1, Gain/1
  Ri/1 -> Switch13/1
  Mux13/1 -> Scope42/1
  Ri4/1 -> Switch13/3
  Product1/1 -> Switch13/2, Mux13/1, Saturation Dynamic/2
  Gain6/1 -> MATLAB Function2/2(Ri), iRt/1
  MATLAB Function2/1(I_batt) -> Gain9/1
  Gain8/1 -> Product/2
  Gain9/1 -> Ibatt1/1
  Memory1/1 -> Product1/2, Scope15/1
  Constant1/1 -> MATLAB Function/8(conDCDC)
  Constant4/1 -> Divide1/2
  Add1/1 -> Scope4/2, Scope8/1, Divide1/3, Product3/2, MATLAB Function/3(V_uc), Voltage/2, Scope12/1
  Divide1/1 -> MATLAB Function/7(convDCDC), Scope1/1
  MATLAB Function/1(Ireq) -> Scope28/1  "Ireq"
  Product2/1 -> Scope3/2, Integrator6/1, Mux1/3, Scope10/3, Add/1
  MATLAB Function1/11(countc) -> ab1/3
  Delay5/1 -> MATLAB Function1/6(cprevb)
  MATLAB Function1/10(countb) -> ab1/2, Delay5/1
  MATLAB Function1/9(counta) -> ab1/1, Delay4/1
  Delay4/1 -> MATLAB Function1/5(cpreva)
  MATLAB Function1/6(a) -> ab/1
  MATLAB Function1/7(b) -> ab/2
  MATLAB Function1/5(count) -> Delay2/1, test/2
  MATLAB Function1/8(test) -> MATLAB Function/6(test), test/1
  MATLAB Function1/4(mo2) -> mod/2
  Delay1/1 -> Scope2/2, MATLAB Function1/2(aprev)
  MATLAB Function1/1(acurr) -> Delay1/1, Scope2/1
  Gain4/1 -> Mux2/2, Scope13/2, MATLAB Function1/1(SoCuc), MATLAB Function/5(SoCuc), Scope57/1  "SOC UC"
  Delay2/1 -> MATLAB Function1/4(cprev)
  Delay3/1 -> Scope2/4, MATLAB Function1/3(bprev)
  MATLAB Function1/2(bcurr) -> Scope2/3, Delay3/1
  MATLAB Function1/3(mo1) -> mod/1
  Memory2/1 -> Product1/1
  Gain/1 -> Scope4/1, Voc/1, MATLAB Function2/1(OCV), Product/1, Scope17/2, Memory2/1, MATLAB Function/2(V_bat), Voltage/1, Product2/1, Divide1/1, Scope8/2  "Voc"
  [vel_or] -> Gain10/1
  Add2/1 -> Scope4/3
  Gain10/1 -> Add2/1
  Constant/1 -> Add2/2
  Product3/1 -> Integrator7/1, Mux1/4, Scope10/4, Add/2
  Subsystem/1(Out1) -> vehicle dynamics/1("Force_FA ")
  SOC/1 -> Mux2/1, Scope13/1, PMG_max/1, PMG_min/1, MATLAB Function/4(SoCbat), Ri4/1, OCV/1, Ri/1, Scope18/2, SoC/1  "SOC bat"
  Mux4/1 -> To Workspace3/1
  Gain14/1 -> Mux4/4, ener Wh2/4
  Gain13/1 -> Mux4/3, ener Wh2/3
  Gain12/1 -> Mux4/2, ener Wh2/2
  Integrator6/1 -> Gain13/1
  Gain15/1 -> Mux4/1, ener Wh2/1
  Integrator4/1 -> Gain15/1
  Integrator7/1 -> Gain14/1
  Mux2/1 -> To Workspace1/1
  Mux1/1 -> To Workspace/1
  Integrator5/1 -> Gain12/1
  Constant5/1 -> Switch1/1, Switch/3
  Switch/1 -> Integrator/1, Scope55/2
  Switch1/1 -> Integrator3/1, Scope55/3
  Integrator/1 -> Gain16/1
  Integrator3/1 -> Gain17/1
  Integrator8/1 -> Gain18/1
  Gain16/1 -> Scope5/1
  Gain17/1 -> Scope5/2
  Gain18/1 -> Scope5/3
  Constant2/1 -> Integrator9/1
  Integrator9/1 -> Scope6/1
  Constant6/1 -> Datasheet Battery/2
  Datasheet Battery/1 -> Scope16/1, Bus Selector/1
  MATLAB Function/3(Ibat) -> Scope7/1, Datasheet Battery/1, Gain8/1, Ibatt1/2, Mux3/1, Memory1/1, Scope11/1, Product2/2, Scope28/3  "I_batt"
  Datasheet Battery/2 -> Scope17/1  "Voltage"
  Bus Selector/1 -> Scope18/1  "<BattSoc>"
  Mux3/1 -> To Workspace4/1

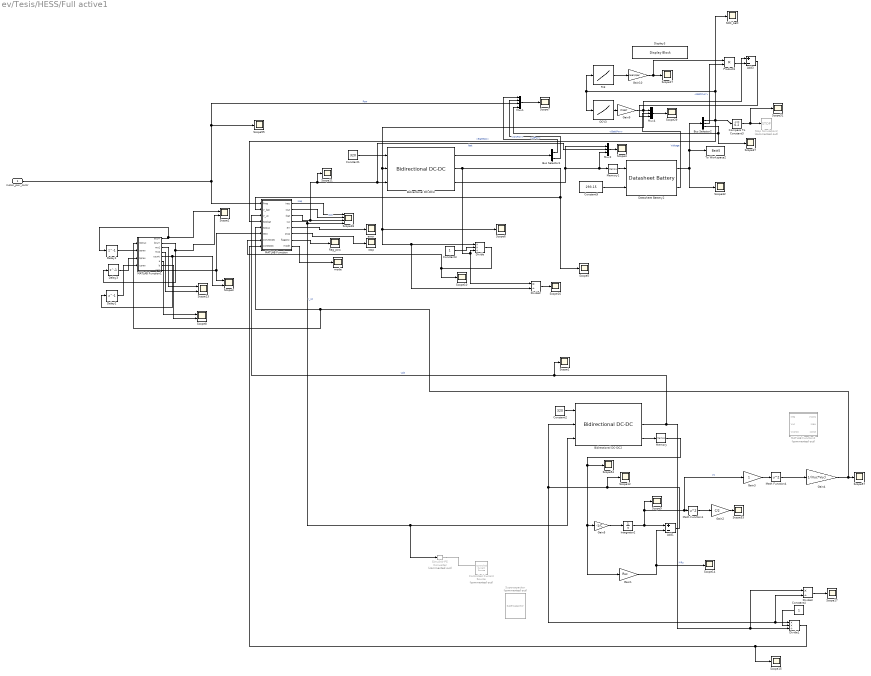
== system ev/Tesis/HESS/Full active1 ==
  motor_pwr_contr : Inport
  Add1 : Sum  Inputs=+-
  Add3 : Sum  Inputs=+-
  Bidirectional DC-DC2 : autolibdcdc/Bidirectional DC-DC  Tc=1/1000  Vinit=320  Plimit=100000  param_loss=Single efficiency measurement  eff=100  v_loss_bp=[0 200 400 600 800 1000]  i_loss_bp=[0 25 50 75 100]  losses_table=[100 100 100 100 100;100 150 200 250 300;100 200 300 400 500;100 250 400 550 700;100 300 500 700 900;100 350 600 850 1100]  v_eff_bp=[200 400 600 800 1000]  i_eff_bp=[25 50 75 100]  efficiency_table=[96.2 98.1 98.7 99;98.1 99 99.4 99.5;98.7 99.4 99.6 99.7;99 99.5 99.7 99.8;99.2 99.6 99.7 99.8]  x_v_bp=[-1000 -800 -600 -400 -200 200 400 600 800 1000]  x_i_bp=[-100 -75 -50 -25 25 50 75 100]  x_losses_mat=[200.400801603196 225.67703109328 200.803212851408 201.612903225806 199.999999999997 200 225 200;160.320641282556 180.541624874624 201.005025125625 202.020202020203 200 200 180 160;180.541624874624 180.722891566267 181.086519114686 197.568389057748 194.999999999999 179.999999999997 180 180;201.005025125625 181.086519114686 202.020202020203 193.67991845056 190 200 179.999999999997 200;202.020202020203 197.568389057748 193.67991845056 197.505197505197 190 190 194.999999999999 200;200 194.999999999999 190 190 197.505197505197 193.67991845056 197.568389057748 202.020202020203;200 179.999999999997 200 190 193.67991845056 202.020202020203 181.086519114686 201.005025125625;180 180 179.999999999997 194.999999999999 197.568389057748 181.086519114686 180.722891566267 180.541624874624;160 180 200 200 202.020202020203 201.005025125625 180.541624874624 160.320641282556;200 225 200 199.999999999997 201.612903225806 200.803212851408 225.67703109328 200.400801603196]  RefBlkName='autolibdcdc/Bidirectional DC-DC'
      settings: SourceProductBaseCode=PW
  Bidirectional DC-DC3 : autolibdcdc/Bidirectional DC-DC  Tc=1/1000  Vinit=320  Plimit=100000  param_loss=Single efficiency measurement  eff=100  v_loss_bp=[0 200 400 600 800 1000]  i_loss_bp=[0 25 50 75 100]  losses_table=[100 100 100 100 100;100 150 200 250 300;100 200 300 400 500;100 250 400 550 700;100 300 500 700 900;100 350 600 850 1100]  v_eff_bp=[200 400 600 800 1000]  i_eff_bp=[25 50 75 100]  efficiency_table=[96.2 98.1 98.7 99;98.1 99 99.4 99.5;98.7 99.4 99.6 99.7;99 99.5 99.7 99.8;99.2 99.6 99.7 99.8]  x_v_bp=[-1000 -800 -600 -400 -200 200 400 600 800 1000]  x_i_bp=[-100 -75 -50 -25 25 50 75 100]  x_losses_mat=[200.400801603196 225.67703109328 200.803212851408 201.612903225806 199.999999999997 200 225 200;160.320641282556 180.541624874624 201.005025125625 202.020202020203 200 200 180 160;180.541624874624 180.722891566267 181.086519114686 197.568389057748 194.999999999999 179.999999999997 180 180;201.005025125625 181.086519114686 202.020202020203 193.67991845056 190 200 179.999999999997 200;202.020202020203 197.568389057748 193.67991845056 197.505197505197 190 190 194.999999999999 200;200 194.999999999999 190 190 197.505197505197 193.67991845056 197.568389057748 202.020202020203;200 179.999999999997 200 190 193.67991845056 202.020202020203 181.086519114686 201.005025125625;180 180 179.999999999997 194.999999999999 197.568389057748 181.086519114686 180.722891566267 180.541624874624;160 180 200 200 202.020202020203 201.005025125625 180.541624874624 160.320641282556;200 225 200 199.999999999997 201.612903225806 200.803212851408 225.67703109328 200.400801603196]  RefBlkName='autolibdcdc/Bidirectional DC-DC'
      settings: SourceProductBaseCode=PW
  Bus Selector1 : BusSelector  OutputSignals=SrcPwr,LdPwr
  Bus Selector2 : BusSelector  OutputSignals=BattSoc,BattCurr,BattPwr
  Compare To Constant3 : simulink/Logic and Bit Operations/Compare To Constant  relop=<=  const=0.2  OutDataTypeStr=boolean
  Constant1 : Constant  Value=320
  Constant2 : Constant  Value=320
  Constant3 : Constant
  Constant4 : Constant
  Constant9 : Constant  Value=293.15
  Controlled Current Source : fl_lib/Electrical/Electrical Sources/Controlled Current Source  Commented=on
  Datasheet Battery2 : autolibdatasheetbattery/Datasheet Battery  CapacityCtrl=Parameter  OutputVlt=Unfiltered  BattChargeMax=Qbat  Em=Voc_BP  CapLUTBp=SOC_BP  RInt=iR_bp  BattTempBp=Temp_bp  CapSOCBp=SOC_BP  Ns=nser  Np=npar  BattCapInit=Qbat*(1-DoD)  Tc=0.01  Vinit=3.3342*nser  RefBlkName='autolibdatasheetbattery/Datasheet Battery'
      settings: SourceProductBaseCode=PW
  Delay1 : Delay  DelayLength=1  InitialCondition=0
  Delay2 : Delay  DelayLength=1  InitialCondition=0
  Delay3 : Delay  DelayLength=1  InitialCondition=0
  Display3 : DisplayBlock  LabelPosition=Hide  Format=short  Transparency=1
  Divide : Product  Inputs=**/
  Divide1 : Product  Inputs=**/
  Divide2 : Product  Inputs=*/
  Divide3 : Product  Inputs=*/
  Gain1 : Gain  Gain=Rsc
  Gain10 : Gain  Gain=nser/npar
  Gain2 : Gain  Gain=C/2
  Gain3 : Gain
  Gain4 : Gain  Gain=1/(Vuc*Vuc)
  Gain5 : Gain  Gain=-1/C
  Gain9 : Gain  Gain=nser
  Integrator2 : Integrator  InitialCondition=Vuc*0.5  UpperSaturationLimit=Vuc  LowerSaturationLimit=Vuc*0
  MATLAB Function : MATLAB Function  TreatAsAtomicUnit=on
  MATLAB Function1 : MATLAB Function  TreatAsAtomicUnit=on
  MATLAB Function2 : MATLAB Function  Commented=on  TreatAsAtomicUnit=on
  Math Function1 : Math  Operator=square  SaturateOnIntegerOverflow=on
  Math Function4 : Math  Operator=square  SaturateOnIntegerOverflow=on
  Memory : Memory
  Memory1 : Memory
  Mux1 : Mux
  Mux2 : Mux  Inputs=3
  Mux4 : Mux  Inputs=3
  OCV3 : Lookup_n-D  NumberOfTableDimensions=1  BreakpointsForDimension1=SOC_BP  Table=Voc_BP  InternalRulePriority=Speed  RndMeth=Simplest  InputSameDT=on
  Product3 : Product
  Ri3 : Lookup_n-D  NumberOfTableDimensions=1  BreakpointsForDimension1=SOC_BP  Table=Ri_BP  InternalRulePriority=Speed  RndMeth=Simplest  InputSameDT=on
  SOC_batt : Scope
  Scope{1,4..7,9..12,14..17,27,29,31..32,37,53..55,57} (22 alike) : Scope
  Scope{2..3,8,13} (4 alike) : Scope  NumInputPorts=2
  Scope28 : Scope  NumInputPorts=4
  Simulink-PS Converter : nesl_utility/Simulink-PS Converter  Commented=on  PhysicalDomain=network_engine_domain  SubClassName=ps_input  LeftPortType=input  RightPortType=output  PseudoPeriodic=off  Frequencies=[]  NoiseDistribution=none  NoiseParameters=[]  Unit=A  AffineConversion=off  FilteringAndDerivatives=provide  SimscapeFilterOrder=1  InputFilterTimeConstant=0.001  UdotUserProvided=0
      settings: SourceProductBaseCode=PW,SS
  Stop Simulation2 : Stop  Commented=on
  Supercapacitor : spsSupercapacitorLib/Supercapacitor  Commented=on  C=99.5  Rdc=8.9e-3  Voltage=48  Ns=18  Np=1  Vinit=0  Temp=25  PresetModel=off  EstParam=off  Nc=1  r=1e-9  epsilon=6.0208e-10  Ich=10  Vstern="[0.161  2.7  7.8]"  Self_dis=on  Ioc=10  Vself="[48  47.8  47.06  44.65]"  demandeplot=off  I="[10  20 100  500]"  Units=sec  Vmax=0  If=0  deltaV=0  alpha=0  sec=0
      settings: SourceProductBaseCode=PS
  To Workspace2 : ToWorkspace  VariableName=Batt5  SaveFormat=Structure With Time  SampleTime=-1
  error : Scope
  flag_pow : Scope
  mode : Scope
  stop : Scope
  wires:
  motor_pwr_contr/1 -> Scope55/1, Mux1/3, MATLAB Function/1(Preq)  "Pow"
  MATLAB Function/3(Ibat) -> Scope11/1, Bidirectional DC-DC3/3, Mux2/2, Scope28/3  "Ibat"
  Constant9/1 -> Datasheet Battery2/2
  Mux4/1 -> Scope29/1
  Datasheet Battery2/1 -> Scope32/1, Bus Selector2/1, To Workspace2/1
  Datasheet Battery2/2 -> Mux4/2  "Voltage"
  Constant1/1 -> Bidirectional DC-DC3/1
  Bus Selector2/2 -> Product3/2  "<BattCurr>"
  Mux1/1 -> Scope7/1
  Product3/1 -> Add3/2
  Bus Selector1/2 -> Mux1/2  "<LdPwr>"
  Gain10/1 -> Product3/1, Scope27/1
  Bus Selector1/1 -> Mux1/1  "<SrcPwr>"
  Mux2/1 -> Scope4/1
  Bus Selector2/1 -> SOC_batt/1, Ri3/1, OCV3/1, MATLAB Function/4(SoCbat), Compare To Constant3/1  "<BattSoc>"
  Add3/1 -> Mux4/3
  Bidirectional DC-DC3/2 -> Divide2/1, Divide/3, Scope5/1, MATLAB Function/2(V_bat)
  Compare To Constant3/1 -> Scope31/1, Stop Simulation2/1
  Gain9/1 -> Scope6/1, Divide/1, Divide2/2, Bidirectional DC-DC3/2, Add3/1, Mux4/1
  Bus Selector2/3 -> Scope37/1, Mux1/4  "<BattPwr>"
  Ri3/1 -> Gain10/1
  Bidirectional DC-DC3/1 -> Bus Selector1/1
  OCV3/1 -> Gain9/1
  Bidirectional DC-DC3/3 -> Mux2/3, Memory1/1, Mux2/1
  MATLAB Function1/1(acurr) -> Delay1/1, Scope2/1
  MATLAB Function1/2(bcurr) -> Delay3/1, Scope2/2
  MATLAB Function/2(Iout) -> Scope28/2  "Iout"
  MATLAB Function/1(Ireq) -> Scope28/1  "Ireq"
  MATLAB Function/5(err) -> error/1
  MATLAB Function/6(stop) -> stop/1
  MATLAB Function/7(flagpow) -> flag_pow/1
  MATLAB Function/8(mode) -> mode/1
  MATLAB Function1/3(mo1) -> Scope13/1
  Delay1/1 -> MATLAB Function1/2(aprev)
  Delay3/1 -> MATLAB Function1/3(bprev)
  MATLAB Function1/5(count) -> Scope3/2, Delay2/1
  MATLAB Function1/4(mo2) -> Scope13/2
  Delay2/1 -> MATLAB Function1/4(cprev)
  MATLAB Function1/6(a) -> Scope8/1
  MATLAB Function1/7(b) -> Scope8/2
  MATLAB Function1/8(test) -> Scope3/1, MATLAB Function/6(test)
  Gain1/1 -> Add1/2, Scope14/1  "i*Rs"
  Gain2/1 -> Scope53/1
  Math Function4/1 -> Gain4/1
  Gain4/1 -> MATLAB Function/5(SoCuc), MATLAB Function1/1(SoCuc), Scope57/1
  Math Function1/1 -> Gain2/1
  Gain5/1 -> Integrator2/1
  Gain3/1 -> Math Function4/1
  Constant2/1 -> Bidirectional DC-DC2/1
  Bidirectional DC-DC2/2 -> Divide3/1, Divide1/3, MATLAB Function/3(V_uc), Scope1/1  "volt"
  MATLAB Function/4(Iuc) -> Simulink-PS Converter/1, Bidirectional DC-DC2/3, Scope28/4  "I_uc"
  Integrator2/1 -> Scope9/1, Gain3/1, Math Function1/1, Add1/1  "Vc"
  Bidirectional DC-DC2/3 -> Memory/1
  Memory/1 -> Gain1/1, Gain5/1, Scope54/1
  Memory1/1 -> Datasheet Battery2/1
  Divide/1 -> Scope10/1, MATLAB Function/7(convDCDC)
  Constant3/1 -> Divide/2
  Constant4/1 -> Divide1/2
  Add1/1 -> Divide3/2, Divide1/1, Bidirectional DC-DC2/2, Scope12/1
  Divide1/1 -> MATLAB Function/8(conDCDC), Scope15/1
  Divide2/1 -> Scope16/1
  Divide3/1 -> Scope17/1
  connections:
  Simulink-PS Converter/RConn1 -- Controlled Current Source/RConn1

== system ev/Tesis/HESS/Full active2 ==
  motor_pwr_contr : Inport
  Add7 : Sum  Inputs=+-
  Bidirectional DC-DC1 : autolibdcdc/Bidirectional DC-DC  Tc=1/1000  Vinit=320  Plimit=100000  param_loss=Single efficiency measurement  eff=95  v_loss_bp=[0 200 400 600 800 1000]  i_loss_bp=[0 25 50 75 100]  losses_table=[100 100 100 100 100;100 150 200 250 300;100 200 300 400 500;100 250 400 550 700;100 300 500 700 900;100 350 600 850 1100]  v_eff_bp=[200 400 600 800 1000]  i_eff_bp=[25 50 75 100]  efficiency_table=[96.2 98.1 98.7 99;98.1 99 99.4 99.5;98.7 99.4 99.6 99.7;99 99.5 99.7 99.8;99.2 99.6 99.7 99.8]  x_v_bp=[-1000 -800 -600 -400 -200 200 400 600 800 1000]  x_i_bp=[-100 -75 -50 -25 25 50 75 100]  x_losses_mat=[200.400801603196 225.67703109328 200.803212851408 201.612903225806 199.999999999997 200 225 200;160.320641282556 180.541624874624 201.005025125625 202.020202020203 200 200 180 160;180.541624874624 180.722891566267 181.086519114686 197.568389057748 194.999999999999 179.999999999997 180 180;201.005025125625 181.086519114686 202.020202020203 193.67991845056 190 200 179.999999999997 200;202.020202020203 197.568389057748 193.67991845056 197.505197505197 190 190 194.999999999999 200;200 194.999999999999 190 190 197.505197505197 193.67991845056 197.568389057748 202.020202020203;200 179.999999999997 200 190 193.67991845056 202.020202020203 181.086519114686 201.005025125625;180 180 179.999999999997 194.999999999999 197.568389057748 181.086519114686 180.722891566267 180.541624874624;160 180 200 200 202.020202020203 201.005025125625 180.541624874624 160.320641282556;200 225 200 199.999999999997 201.612903225806 200.803212851408 225.67703109328 200.400801603196]  RefBlkName='autolibdcdc/Bidirectional DC-DC'
      settings: SourceProductBaseCode=PW
  Constant15 : Constant  Value=320
  Current_calc4 : Product  Inputs=/*
  Gain : Gain  Gain=nser
  Gain1 : Gain  Gain=nser/npar
  Gain11 : Gain  Gain=(Qbat*VinBat*nser*npar)
  Gain2 : Gain  Gain=1/(Qbat*VinBat*nser*npar*3600)
  Gain20 : Gain  Gain=Rsc
  Gain22 : Gain  Gain=C/2
  Gain23 : Gain
  Gain24 : Gain  Gain=1/(Vuc*Vuc)
  Gain25 : Gain  Gain=-1/C
  Ibatt1 : Scope
  Integrator2 : Integrator
  Integrator6 : Integrator  InitialCondition=Vuc*1
  MATLAB Function : MATLAB Function  TreatAsAtomicUnit=on
  MATLAB Function1 : MATLAB Function  TreatAsAtomicUnit=on
  MATLAB Function2 : MATLAB Function  TreatAsAtomicUnit=on
  Math Function2 : Math  Operator=square  SaturateOnIntegerOverflow=on
  Math Function3 : Math  Operator=square  SaturateOnIntegerOverflow=on
  Mux14 : Mux  Inputs=2
  OCV : Lookup_n-D  NumberOfTableDimensions=1  BreakpointsForDimension1=SOC_BP  Table=Voc_BP  InternalRulePriority=Speed  RndMeth=Simplest  InputSameDT=on
  Pow1 : Scope
  Product : Product
  Ri : Lookup_n-D  NumberOfTableDimensions=1  BreakpointsForDimension1=SOC_BP  Table=Ri_BP  InternalRulePriority=Speed  RndMeth=Simplest  InputSameDT=on
  Ri4 : Lookup_n-D  NumberOfTableDimensions=1  BreakpointsForDimension1=SOC_BP  Table=Ri_BP  InternalRulePriority=Speed  RndMeth=Simplest  InputSameDT=on
  SOC : Integrator  InitialCondition=(1-DoD)
  Scope{,1,45,53..55,57..58,60} (9 alike) : Scope
  Scope28 : Scope  NumInputPorts=2
  SoC : Scope
  Switch13 : Switch  Criteria=u2 > Threshold
  Vo : Scope
  Vo1 : Scope
  Voc : Scope
  ener Wh : Scope
  iR : Scope
  iRt : Scope
  Info : Outport
  wires:
  motor_pwr_contr/1 -> Scope55/1, MATLAB Function/1(P_req)  "Pow"
  MATLAB Function/3(err) -> Scope/1
  Gain2/1 -> Integrator2/1, SOC/1
  SOC/1 -> OCV/1, Ri/1, Ri4/1, SoC/1  "SOC"
  MATLAB Function2/1(Vb) -> Mux14/1
  Integrator2/1 -> Gain11/1
  Gain11/1 -> ener Wh/1
  Gain1/1 -> MATLAB Function2/1(Ri), MATLAB Function1/2(Ri), iRt/1
  MATLAB Function1/1(I_batt) -> Ibatt1/1, MATLAB Function2/2(Ib), Product/2
  Product/1 -> Pow1/1, Gain2/1
  Ri4/1 -> Switch13/3
  Ri/1 -> Switch13/1
  Switch13/1 -> Gain1/1, iR/1
  Gain/1 -> MATLAB Function1/1(OCV), Product/1, Mux14/2, Voc/1
  MATLAB Function/1(P_batt) -> Vo1/1, MATLAB Function1/3(P), Switch13/2, MATLAB Function2/3(Pmot), Scope28/1
  OCV/1 -> Vo/1, Gain/1
  Mux14/1 -> Scope45/1
  Current_calc4/1 -> Bidirectional DC-DC1/3, Gain20/1, Scope58/1  "I_uc"
  Bidirectional DC-DC1/3 -> Gain25/1
  Gain24/1 -> Scope57/1
  Gain25/1 -> Integrator6/1  "i/C"
  Bidirectional DC-DC1/2 -> Current_calc4/1
  Gain22/1 -> Scope53/1
  Math Function2/1 -> Gain22/1
  Constant15/1 -> Bidirectional DC-DC1/1
  Gain20/1 -> Add7/2, Scope60/1  "i*Rs"
  MATLAB Function/2(P_uc) -> Scope1/1, Current_calc4/2, Scope28/2  "Pow"
  Gain23/1 -> Math Function3/1
  Bidirectional DC-DC1/1 -> Info/1
  Add7/1 -> Scope54/1, Bidirectional DC-DC1/2
  Math Function3/1 -> Gain24/1
  Integrator6/1 -> Gain23/1, Math Function2/1, Add7/1  "Vc"
